simulink model "throttle"  (R2016b)
settings: Solver=VariableStepAuto  StartTime=0.0  StopTime=20  RelTol=1e-3
undefined symbols (not defined in the file): sigbuilder_block
libraries: simulink x1
settings Model: Creator=nguyenquoctruong  LastModifiedBy=nguyenquoctruong

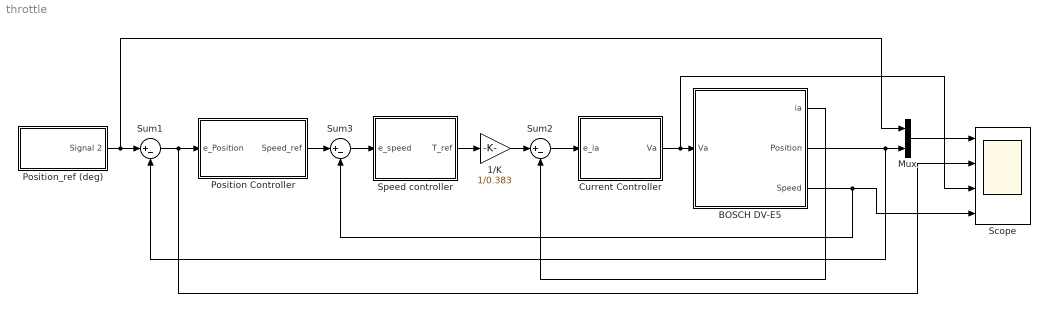
== system throttle ==
  1/K : Gain  Gain=1/0.383
  BOSCH DV-E5 : Subsystem  mask{Ra=1.15, K=0.383, Jeq=0.0021, La=1.5*(10^-3), beq=0.0088, Ks=0.087, Tpl=0.396, Tf=0.284}
      mask prompts: Ra "Ra(Ohm)"; K "K(V.s/rad)"; Jeq "Jeq(kgm^2)"; La "La(H)"; beq "beq(Nm.s.rad^-1)"; Ks "Ks(N.m/rad)"; Tpl "Tpl(N.m)"; Tf "Tf(N.m)"
  Current Controller : Subsystem  mask{Kp=5, Ki=0.004, Vmax=12}
      mask prompts: Vmax "Vmax(V)"
  Mux : Mux  Inputs=2
  Position Controller : Subsystem  mask{Kp=3, Ki=0.01, Speedmax=234}
      mask prompts: Speedmax "Speedmax(rpm)"
  Position_ref (deg) : Subsystem  Tag=STV Subsys  LoadFcn=sigbuilder_block('load');  StartFcn=sigbuilder_block('start');  StopFcn=sigbuilder_block('stop');  ClipboardFcn=sigbuilder_block('clipboard');  mask(Sigbuilder block){tuvar=[0:10]}
      mask help: Simulink:masks:SigbuilderBlock_MD
      mask init:
      | if ~strcmp(get_param(bdroot(gcbh),'SimulationStatus'),'stopped') tuvar = sigbuilder_block('maskInit'); end
      settings: CopyFcn=sigbuilder_block('copy');  DeleteFcn=sigbuilder_block('delete');  ModelCloseFcn=sigbuilder_block('modelClose');  PreSaveFcn=sigbuilder_block('preSave');  PauseFcn=sigbuilder_block('pause');  ContinueFcn=sigbuilder_block('continue');  NameChangeFcn=sigbuilder_block('namechange');  OpenFcn=sigbuilder_block('open',[196.5 100.5 550.5 359.25 ]);  CloseFcn=sigbuilder_block('close');
      mask Display: plot(0, 0, 100, 100,[2, 2, 32, 32, 2], [68, 8, 8, 68, 68],[32, 2], [38, 38], [32, 19, 2],[53, 60, 44], [32, 17, 17, 2],[16, 16, 31, 31]);txt = getActiveGroup(gcbh);text(2, 100, txt,'verticalAlignment', 'top');
  Scope : Scope  NumInputPorts=4
  Speed controller : Subsystem  mask{Kp=10, Ki=1, Tmax=3.5}
      mask prompts: Tmax "Tmax(Nm)"
  Sum1 : Sum  Inputs=|+-
  Sum2 : Sum  Inputs=|+-
  Sum3 : Sum  Inputs=|+-
  wires:
  BOSCH DV-E5/1(ia) -> Sum2/2
  1/K/1 -> Sum2/1
  Sum1/1 -> Scope/2, Position Controller/1(e_Position)
  BOSCH DV-E5/3("Speed ") -> Sum3/2, Scope/4
  Position Controller/1("Speed_ref ") -> Sum3/1
  Speed controller/1("T_ref ") -> 1/K/1
  Sum3/1 -> Speed controller/1(e_speed)
  Sum2/1 -> Current Controller/1(e_ia)
  Current Controller/1("Va ") -> Scope/3, BOSCH DV-E5/1("Va ")
  Mux/1 -> Scope/1
  Position_ref (deg)/1(Signal 2) -> Mux/1, Sum1/1
  BOSCH DV-E5/2(Position) -> Mux/2, Sum1/2

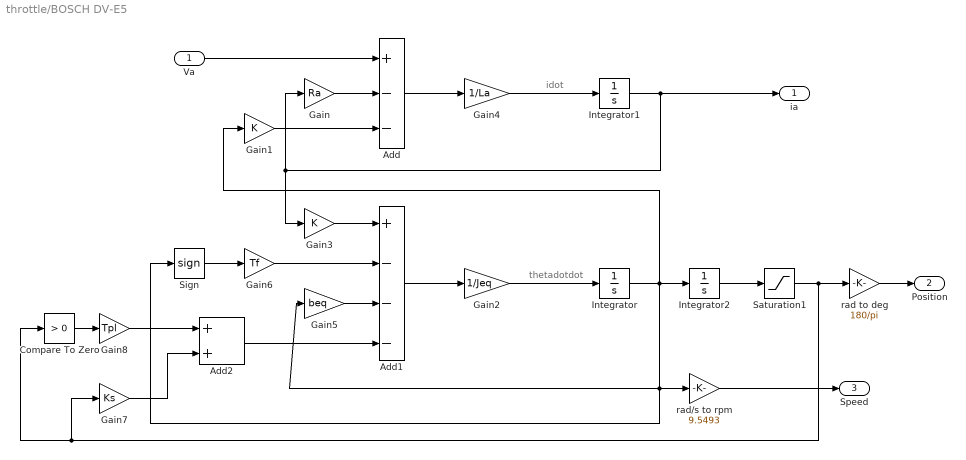
== system throttle/BOSCH DV-E5 ==
  note: idot
  note: thetadotdot
  "Va " : Inport
  Add : Sum  Inputs=+--
  Add1 : Sum  Inputs=+---
  Add2 : Sum
  Compare To Zero : simulink/Logic and Bit Operations/Compare To Zero  relop=>  OutDataTypeStr=uint8
  Gain : Gain  Gain=Ra
  Gain1 : Gain  Gain=K
  Gain2 : Gain  Gain=1/Jeq
  Gain3 : Gain  Gain=K
  Gain4 : Gain  Gain=1/La
  Gain5 : Gain  Gain=beq
  Gain6 : Gain  Gain=Tf
  Gain7 : Gain  Gain=Ks
  Gain8 : Gain  Gain=Tpl
  Integrator : Integrator
  Integrator1 : Integrator
  Integrator2 : Integrator
  Saturation1 : Saturate  UpperLimit=pi/2  LowerLimit=0
  Sign : Signum
  rad to deg : Gain  Gain=180/pi
  rad/s to rpm : Gain  Gain=9.5493
  ia : Outport
  Position : Outport  Port=2
  "Speed " : Outport  Port=3
  wires:
  Sign/1 -> Gain6/1
  Add2/1 -> Add1/4
  Gain7/1 -> Add2/2
  Gain6/1 -> Add1/2
  Integrator/1 -> Gain1/1, Integrator2/1, Sign/1, Gain5/1, rad/s to rpm/1
  Gain5/1 -> Add1/3
  Integrator1/1 -> Gain3/1, Gain/1, ia/1
  Gain2/1 -> Integrator/1
  Add1/1 -> Gain2/1
  Add/1 -> Gain4/1
  Gain4/1 -> Integrator1/1
  "Va "/1 -> Add/1
  Gain3/1 -> Add1/1
  Gain1/1 -> Add/3
  Gain/1 -> Add/2
  Integrator2/1 -> Saturation1/1
  rad to deg/1 -> Position/1
  Gain8/1 -> Add2/1
  Compare To Zero/1 -> Gain8/1
  rad/s to rpm/1 -> "Speed "/1
  Saturation1/1 -> rad to deg/1, Compare To Zero/1, Gain7/1

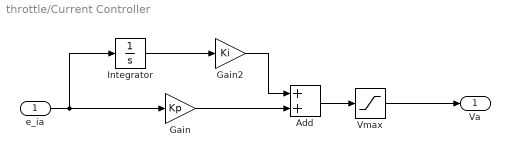
== system throttle/Current Controller ==
  e_ia : Inport
  Add : Sum
  Gain : Gain  Gain=Kp
  Gain2 : Gain  Gain=Ki
  Integrator : Integrator
  Vmax : Saturate  UpperLimit=Vmax  LowerLimit=-Vmax
  "Va " : Outport
  wires:
  Integrator/1 -> Gain2/1
  e_ia/1 -> Integrator/1, Gain/1
  Gain2/1 -> Add/1
  Add/1 -> Vmax/1
  Vmax/1 -> "Va "/1
  Gain/1 -> Add/2

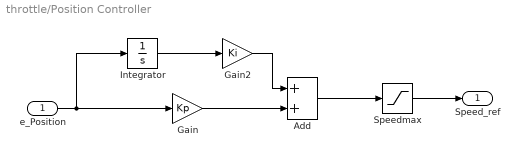
== system throttle/Position Controller ==
  e_Position : Inport
  Add : Sum
  Gain : Gain  Gain=Kp
  Gain2 : Gain  Gain=Ki
  Integrator : Integrator
  Speedmax : Saturate  UpperLimit=Speedmax  LowerLimit=-Speedmax
  "Speed_ref " : Outport
  wires:
  Add/1 -> Speedmax/1
  Gain2/1 -> Add/1
  Gain/1 -> Add/2
  Integrator/1 -> Gain2/1
  Speedmax/1 -> "Speed_ref "/1
  e_Position/1 -> Gain/1, Integrator/1

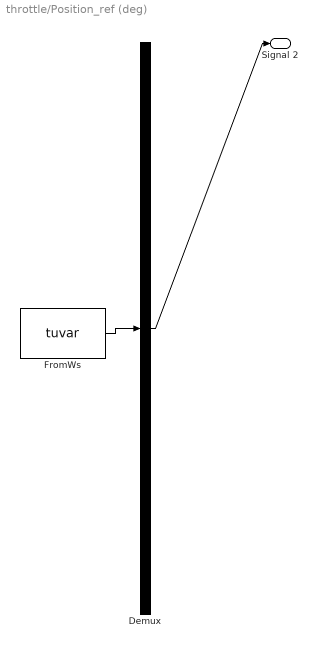
== system throttle/Position_ref (deg) ==
  Demux : Demux  Tag=STV Demux  Outputs=1
  FromWs : FromWorkspace  Tag=STV FromWs  VariableName=tuvar  SampleTime=0
      SigBuilderData=|
      | common.afterFinalStr = 'Extrapolate'
      | common.sampleTime = 0
      | dataSet.timeRange = [0 20]
      | dataSet.name = 'Group 1'
      | sbobj.Groups.Name = 'Group 1'
      | sbobj.Groups.Signals.Name = 'Signal 2'
      | sbobj.Groups.Signals.XData = [0 1 1 5 5 10 12 12 18 18 20]
      | sbobj.Groups.Signals.YData = [0 0 30 30 90 90 90 60 60 0 0]
      | sbobj.Groups.TimeRange = [0 20]
  Signal 2 : Outport  Tag=STV Outport
  wires:
  FromWs/1 -> Demux/1
  Demux/1 -> Signal 2/1

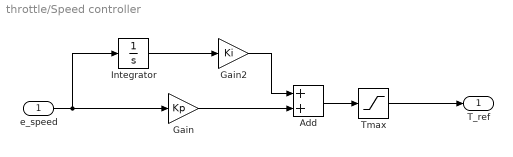
== system throttle/Speed controller ==
  e_speed : Inport
  Add : Sum
  Gain : Gain  Gain=Kp
  Gain2 : Gain  Gain=Ki
  Integrator : Integrator
  Tmax : Saturate  UpperLimit=Tmax  LowerLimit=-Tmax
  "T_ref " : Outport
  wires:
  Gain/1 -> Add/2
  Tmax/1 -> "T_ref "/1
  Add/1 -> Tmax/1
  Gain2/1 -> Add/1
  e_speed/1 -> Gain/1, Integrator/1
  Integrator/1 -> Gain2/1
